simulink model "IPMSMTorqueBasedLoad_PQ"  (R2022a)
settings: Solver=FixedStepDiscrete  StartTime=0.0  StopTime=0.25  FixedStep=Ts  RelTol=1e-3  EnableMultiTasking=on
PreLoadFcn:
  | ee_ipmsm_torque_control_data;
  | Ts = 5e-6;
StopFcn:
  | ee_addSimlogTimeStamp(bdroot)
undefined symbols (not defined in the file or in its folder): Ld, Lq, p, psim, VDC_VECT
libraries: nesl_utility x13, fl_lib x9, ee_lib x5, eeTransforms x2, eePmsmCurrentController x1, simulink x1, eeGeneralControl x1, eePmsmCurrentReferenceGen x1, eePmsmTorqueEstimator x1, eePwmGeneratorTwoLevel x1, SignalEditorBlockLib x1
CloseFcn:
  | try,close(h1_ee_ipmsm_torque_control),end
  | clear h1_ee_ipmsm_torque_control
  | try,close(h2_ee_ipmsm_torque_control),end
  | clear h2_ee_ipmsm_torque_control
  | try,close(h3_ee_ipmsm_torque_control),end
  | clear h3_ee_ipmsm_torque_control
  | try,close(h4_ee_ipmsm_torque_control),end
  | clear h4_ee_ipmsm_torque_control
  | 
  | 
  | clear simlog_ee_ipmsm_torque_control
  | clear logsout_ee_ipmsm_torque_control
  | 
  | 
  | clear Pmax Tmax p psim Ld Lq L0 Rs Jm
  | clear Cdc Vnom V1 AH0
  | clear Ts fsw Tsi Kp_id Ki_id Kp_iq Ki_iq
  | clear numd_id dend_id numd_iq dend_iq
  | clear ID_MAP IQ_MAP RPM_VECT TQ_VECT VDC_VECT
Description:
  | IPMSM Torque Control
settings Model: Creator=The MathWorks, Inc.  LastModifiedBy=jvansick
settings SolverCC: AlgebraicLoopSolver=TrustRegion  MaxZcPerStep=1
settings DataIOCC: MaxDataPoints=210000  ReturnWorkspaceOutputs=off  SignalLoggingName=logsout_ee_ipmsm_torque_control
settings OptimizationCC: LifeSpan=inf
settings DebuggingCC: UnderspecifiedInitializationDetection=Classic  MergeDetectMultiDrivingBlocksExec=none  UnconnectedInputMsg=warning  UnconnectedOutputMsg=warning  UnconnectedLineMsg=warning  SFUnexpectedBacktrackingDiag=warning  SFNoUnconditionalDefaultTransitionDiag=warning  SFExecutionAtInitializationDiag=none  SFMachineParentedDataDiag=warning  ArithmeticOperatorsInVariantConditions=warning
settings SFSimCC: SimUseLocalCustomCode=off  CustomCodeUndefinedFunction=UseInterfaceOnly
settings RTWCC: RTWUseLocalCustomCode=off  DLArmComputeVersion=19.05
settings CodeAppCC: StateflowObjectComments=on
settings GRTTargetCC: TargetLangStandard=C89/C90 (ANSI)
settings ConfigComp: CovMetricSettings=dw  CovSaveCumulativeToWorkspaceVar=on  CovSaveSingleToWorkspaceVar=on  CovExternalEMLEnable=off
settings SimscapeCC: SimscapeNormalizeSystem=off  SimscapeLogType=all  SimscapeLogSimulationStatistics=on  SimscapeLogName=simlog_ee_ipmsm_torque_control  SimscapeLogDataHistory=210000

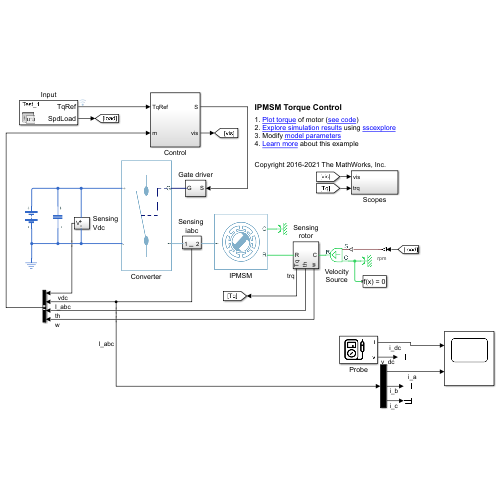
[thumbnail: Simulink's stored preview of the top-level diagram]
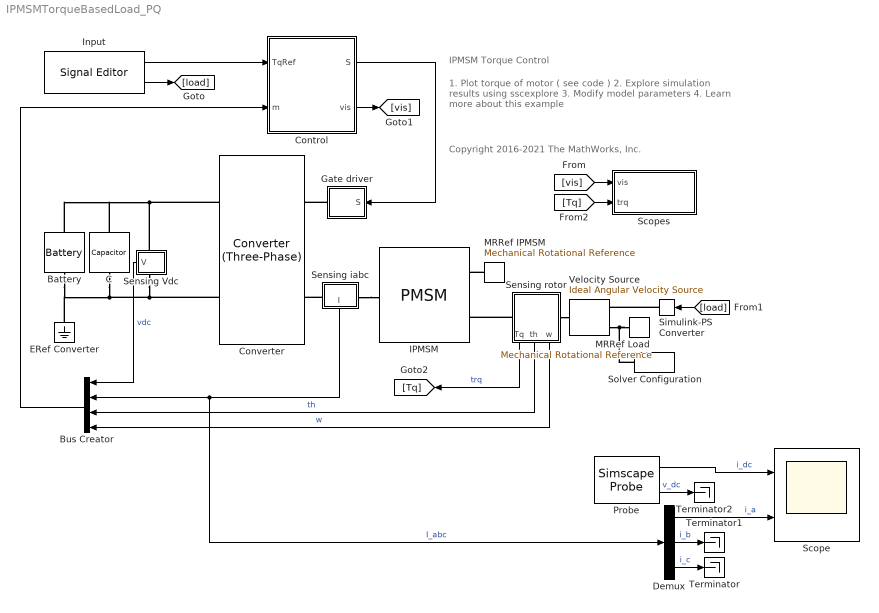
== system IPMSMTorqueBasedLoad_PQ ==
  note: IPMSM Torque Control
  note: 1. Plot torque of motor ( see code )
      | 2. Explore simulation results using sscexplore
      | 3. Modify model parameters
      | 4. Learn more about this example
  note: Copyright 2016-2021 The MathWorks, Inc.
  Battery : ee_lib/Sources/Battery  Vnom=Vnom V  prm_dir=1  R1_dis=2 Ohm  R1_ch=2 Ohm  R1=0.001 Ohm  prm_AH=1  AH=300 hr*A  V1=V1 V  AH1=100 hr*A  prm_R2=1  R2=2000 Ohm  prm_dyn=1  Rp1=0.005 Ohm  tau1=30 s  Rp2=0.005 Ohm  tau2=30 s  Rp3=0.005 Ohm  tau3=30 s  Rp4=0.005 Ohm  tau4=30 s  Rp5=0.005 Ohm  tau5=30 s  prm_fade=1  N_fade=100  AH_fade=45 hr*A  R1_fade=2.02 Ohm  R1_ch_fade=2.02 Ohm  V1_fade=10.35 V  prm_age=1  prm_age_OCV=1  OCV_age=0.9  SOC_age=60  delta_time_age_vec=[0] d  temperature_age_vec=[273] K  OCV_scaling_age=2.2134e6  OCV_offset_age=1.632e6  temp_exp_age=0.515833569 V  t_exp_age=0.75  i_specify=off  i_priority=None  i=0 A  i_nominal_specify=off  i_nominal_unit=A  i_nominal_value=1  v_specify=off  v_priority=None  v=0 V  v_nominal_specify=off  v_nominal_unit=V  v_nominal_value=1  charge_specify=on  charge_priority=High  charge=AH0 hr*A  charge_nominal_specify=off  charge_nominal_unit=hr*A  charge_nominal_value=1  num_cycles_specify=off  num_cycles_priority=High  num_cycles=0  num_cycles_nominal_specify=off  num_cycles_nominal_unit=1  num_cycles_nominal_value=1  Tmeas=298.15 K  Tmeas_age=298.15 K  Vnom_T2=12 V  R1_T2=2.2 Ohm  R1_T2_dis=2.2 Ohm  R1_T2_ch=2.2 Ohm  V1_T2=11.4 V  R2_T2=2200 Ohm  Rp1_T2=0.005 Ohm  tau1_T2=30 s  Rp2_T2=0.005 Ohm  tau2_T2=30 s  Rp3_T2=0.005 Ohm  tau3_T2=30 s  Rp4_T2=0.005 Ohm  tau4_T2=30 s  Rp5_T2=0.005 Ohm  tau5_T2=30 s  Tmeas2=273.15 K  thermal_mass=30000 J/K  temperature_specify=off  temperature_priority=High  temperature=298.15 K  temperature_nominal_specify=off  temperature_nominal_unit=K  temperature_nominal_value=1
  Bus Creator : BusCreator  Inputs=4
  C : fl_lib/Electrical/Electrical Elements/Capacitor  c=Cdc F  r=1e-6 Ohm  g=0 1/Ohm  i_specify=off  i_priority=None  i=0 A  i_nominal_specify=off  i_nominal_unit=A  i_nominal_value=1  v_specify=off  v_priority=None  v=0 V  v_nominal_specify=off  v_nominal_unit=V  v_nominal_value=1  vc_specify=on  vc_priority=None  vc=Vnom V  vc_nominal_specify=off  vc_nominal_unit=V  vc_nominal_value=1
      settings: SourceProductBaseCode=PW,SS,VE
  Control : Subsystem
  Converter : ee_lib/Semiconductors & Converters/Converters/Converter (Three-Phase)  port_option=ee.enum.threePhasePort.composite  device_type=3  Vf=0.8 V  Ron=0.001 Ohm  Rds=0.001 Ohm  Goff=1e-5 1/Ohm  Vgt=1 V  Vgt_off=-1 V  Ih=1 A  Vth=0.5 V  diode_param=2  diode_Vf=0.8 V  diode_Ron=0.001 Ohm  diode_Goff=1e-5 1/Ohm  diode_C=50 nF  diode_iRM=-235 A  diode_iF=300 A  diode_idot=-50 A/us  diode_trr_param=1  diode_trr_factor=3  diode_trr=15 us  diode_Qrr=1.5e+3 s*uA  snubber_type=0  Cs=1e-7 F  Rs=0.1 Ohm
      settings: SourceProductBaseCode=PS
  Demux : Demux  Outputs=3
  ERef Converter : fl_lib/Electrical/Electrical Elements/Electrical Reference
      settings: SourceProductBaseCode=PW,SS,VE
  Gate driver : Subsystem
  IPMSM : ee_lib/Electromechanical/Permanent Magnet/PMSM  port_option=ee.enum.threePhasePort.composite  winding_type=ee.enum.statorconnection.wye  machine_param=ee.enum.pmsm.parameterization.constant  nPolePairs=p  pmflux_param=ee.enum.pmflux.fluxlinkage  pm_flux_linkage=psim Wb  torque_constant=0.18 N*m/A  back_emf_constant=0.18 V/(rad/s)  stator_param=ee.enum.statorparam.LdLqL0  Ld=Ld H  Lq=Lq H  idVec=[-200, 0, 200] A  iqVec=[-200, 0, 200] A  LdMatrix=0.0002 * ones(3, 3) H  LqMatrix=0.0002 * ones(3, 3) H  PmMatrix=0.1 * ones(3, 3) Wb  ktMatrix=0.18 * ones(3, 3) N*m/A  keMatrix=0.18 * ones(3, 3) V/(rad/s)  L0=L0 H  Ls=0.0002 H  Lm=0.00002 H  Ms=0.00002 H  Rs=Rs Ohm  zero_sequence=ee.enum.park.zerosequence.exclude  axes_param=ee.enum.rotorangle.qaxis  loss_param=ee.enum.ironloss.none  losses_oc=[0, 0, 0] W  losses_sc=[0, 0, 0] W  f_losses=60 Hz  Isc_losses=95 A  J=0 kg*m^2  lam=0 N*m/(rad/s)  i_d_specify=off  i_d_priority=None  i_d=0 A  i_d_nominal_specify=off  i_d_nominal_unit=A  i_d_nominal_value=1  i_q_specify=off  i_q_priority=None  i_q=0 A  i_q_nominal_specify=off  i_q_nominal_unit=A  i_q_nominal_value=1  torque_specify=off  torque_priority=None  torque=0 N*m  torque_nominal_specify=off  torque_nominal_unit=N*m  torque_nominal_value=1  angular_velocity_specify=on  angular_velocity_priority=None  angular_velocity=0 rad/s  angular_velocity_nominal_specify=off  angular_velocity_nominal_unit=rpm  angular_velocity_nominal_value=1  angular_position_specify=on  angular_position_priority=High  angular_position=0 rad  angular_position_nominal_specify=off  angular_position_nominal_unit=deg  angular_position_nominal_value=1  alpha=3.93e-3 1/K  alpha_flux=-0.001 1/K  Tmeas=298.15 K  stator_thermal_mass=100 J/K  rotor_thermal_mass=200 J/K  Rm_percent_rotor=90  Rd_percent_rotor=30  temperatureA_specify=off  temperatureA_priority=High  temperatureA=25 degC  temperatureA_nominal_specify=off  temperatureA_nominal_unit=degC  temperatureA_nominal_value=1  temperatureB_specify=off  temperatureB_priority=High  temperatureB=25 degC  temperatureB_nominal_specify=off  temperatureB_nominal_unit=degC  temperatureB_nominal_value=1  temperatureC_specify=off  temperatureC_priority=High  temperatureC=25 degC  temperatureC_nominal_specify=off  temperatureC_nominal_unit=degC  temperatureC_nominal_value=1  temperatureR_specify=off  temperatureR_priority=High  temperatureR=25 degC  temperatureR_nominal_specify=off  temperatureR_nominal_unit=degC  temperatureR_nominal_value=1
      settings: InternalSimscapePortConfiguration="{\"Bottom\":[],\"Left\":[{\"id\":\"N\",\"label\":\"~\",\"type\":\"foundation.electrical.three_phase\"}],\"Right\":[{\"id\":\"R\",\"label\":\"R\",\"type\":\"foundation.mechanical.rotational.rotational\"},{\"id\":\"C\",\"label\":\"C\",\"type\":\"foundation.mechanical.rotational.rotational\"}],\"Top\":[]}"
  Input : SignalEditorBlockLib/Signal Editor  FileName=ee_ipmsm_torque_control_Input.mat  ActiveScenario=Test_1  ActiveSignal=TqRef  IsBus=off  OutputBusObjectStr=Bus: BusObject  SampleTime=0  Interpolate=off  ZeroCross=off  OutputAfterFinalValue=Setting to zero  Unit=inherit  PreserveSignalName=on
  MRRef IPMSM : fl_lib/Mechanical/Rotational Elements/Mechanical Rotational Reference
      settings: SourceProductBaseCode=PW,SS,VE
  MRRef Load : fl_lib/Mechanical/Rotational Elements/Mechanical Rotational Reference
      settings: SourceProductBaseCode=PW,SS,VE
  Probe : SimscapeProbe  BoundBlock=1058  Variables={i, v}
  Scope : Scope  NumInputPorts=2
  Scopes : Subsystem
      settings: PortSchema="{\"entries\":[{\"content\":{\"sides\":[{\"content\":{\"connectorIds\":[]},\"type\":\"ConnectorPlacement.EquallySpacedRectSide\",\"uuid\":\"a560794c-8dec-4526-a26c-129716e1b993\"},{\"content\":{\"connectorIds\":[\"In1\",\"In2\"],\"side\":\"RIGHT\"},\"type\":\"ConnectorPlacement.EquallySpacedRectSide\",\"uuid\":\"247ce755-40a5-4621-9d40-790612a7d15c\"},{\"content\":{\"connectorIds\":[],\"side\":\"TOP\"},\"type\":\"ConnectorPlacement.EquallySpacedRectSide\",\"uuid\":\"3a3e49bb-cf70-44be-b36a-46c371f23d10\"}]},\"type\":\"ConnectorPlacement.EquallySpacedConnector\",\"uuid\":\"881be24b-a5bc-43c9-adfc-ce8dee76105e\"}],\"packageUris\":[\"http://schema.mathworks.com/mf0/Connector/R2020b\"],\"version\":\"1.0\"}"
  Sensing Vdc : Subsystem
      settings: PortSchema="{\"entries\":[{\"content\":{\"sides\":[{\"content\":{\"connectorIds\":[\"LConn1\"]},\"type\":\"ConnectorPlacement.EquallySpacedRectSide\",\"uuid\":\"bc3757cc-4537-444e-89af-7b7d8c8c1fa7\"},{\"content\":{\"connectorIds\":[\"RConn1\"],\"side\":\"RIGHT\"},\"type\":\"ConnectorPlacement.EquallySpacedRectSide\",\"uuid\":\"908bf4c4-26f6-4d8a-bcf8-68236027f5f8\"},{\"content\":{\"connectorIds\":[\"Out1\"],\"side\":\"TOP\"},\"type\":\"ConnectorPlacement.EquallySpacedRectSide\",\"uuid\":\"33f228db-ba47-4718-96dc-a72de309ae8c\"},{\"content\":{\"connectorIds\":[],\"side\":\"BOTTOM\"},\"type\":\"ConnectorPlacement.EquallySpacedRectSide\",\"uuid\":\"d9b66c7e-0954-4c47-8bcc-77bf13ff573c\"}]},\"type\":\"ConnectorPlacement.EquallySpacedConnector\",\"uuid\":\"345f3578-0572-4e64-b2f3-84728129a12d\"}],\"packageUris\":[\"http://schema.mathworks.com/mf0/Connector/R2020b\"],\"version\":\"1.0\"}"
  Sensing rotor : Subsystem
      settings: PortSchema="{\"entries\":[{\"content\":{\"sides\":[{\"content\":{\"connectorIds\":[\"LConn1\"]},\"type\":\"ConnectorPlacement.EquallySpacedRectSide\",\"uuid\":\"bc3757cc-4537-444e-89af-7b7d8c8c1fa7\"},{\"content\":{\"connectorIds\":[\"RConn1\"],\"side\":\"RIGHT\"},\"type\":\"ConnectorPlacement.EquallySpacedRectSide\",\"uuid\":\"908bf4c4-26f6-4d8a-bcf8-68236027f5f8\"},{\"content\":{\"connectorIds\":[],\"side\":\"TOP\"},\"type\":\"ConnectorPlacement.EquallySpacedRectSide\",\"uuid\":\"33f228db-ba47-4718-96dc-a72de309ae8c\"},{\"content\":{\"connectorIds\":[\"Out1\",\"Out2\",\"Out3\"],\"side\":\"BOTTOM\"},\"type\":\"ConnectorPlacement.EquallySpacedRectSide\",\"uuid\":\"5b763560-fcc9-460b-9ba7-46235112184c\"}]},\"type\":\"ConnectorPlacement.EquallySpacedConnector\",\"uuid\":\"345f3578-0572-4e64-b2f3-84728129a12d\"}],\"packageUris\":[\"http://schema.mathworks.com/mf0/Connector/R2020b\"],\"version\":\"1.0\"}"
  Sensing iabc : Subsystem
      settings: PortSchema="{\"entries\":[{\"content\":{\"sides\":[{\"content\":{\"connectorIds\":[\"LConn1\"]},\"type\":\"ConnectorPlacement.EquallySpacedRectSide\",\"uuid\":\"bc3757cc-4537-444e-89af-7b7d8c8c1fa7\"},{\"content\":{\"connectorIds\":[\"RConn1\"],\"side\":\"RIGHT\"},\"type\":\"ConnectorPlacement.EquallySpacedRectSide\",\"uuid\":\"908bf4c4-26f6-4d8a-bcf8-68236027f5f8\"},{\"content\":{\"connectorIds\":[],\"side\":\"TOP\"},\"type\":\"ConnectorPlacement.EquallySpacedRectSide\",\"uuid\":\"33f228db-ba47-4718-96dc-a72de309ae8c\"},{\"content\":{\"connectorIds\":[\"Out1\"],\"side\":\"BOTTOM\"},\"type\":\"ConnectorPlacement.EquallySpacedRectSide\",\"uuid\":\"3b1d40a5-3c80-431c-8111-df754e0c502b\"}]},\"type\":\"ConnectorPlacement.EquallySpacedConnector\",\"uuid\":\"345f3578-0572-4e64-b2f3-84728129a12d\"}],\"packageUris\":[\"http://schema.mathworks.com/mf0/Connector/R2020b\"],\"version\":\"1.0\"}"
  Simulink-PS Converter : nesl_utility/Simulink-PS Converter  PhysicalDomain=network_engine_domain  SubClassName=ps_input  LeftPortType=input  RightPortType=output  PseudoPeriodic=off  Frequencies=[]  NoiseDistribution=none  NoiseParameters=[]  Unit=rpm  AffineConversion=off  FilteringAndDerivatives=zero  SimscapeFilterOrder=1  InputFilterTimeConstant=0.001  UdotUserProvided=1
      settings: SourceProductBaseCode=SS,PW,VE
  Solver Configuration : nesl_utility/Solver Configuration  PhysicalDomain=network_engine_domain  SubClassName=solver  LeftPortType=input  RightPortType=generic  Tones=[]  Harmonics=[]  SimulateNoise=off  Profile=off  UseLocalSampling=off  EnableSwitchedLinearOptims=on  FrequencyDomain=off  UseCCode=off  RelTol=0.001  AbsTol=1e-06  MinStep=1e-09  ToWorkspace=off  RevertToSquareIcSolve=off  NumHomotopyIterations=100  PhasorMode=off  PhasorModeNumHarmonics=1  IndexReductionMethod=DerivativeReplacement  DoDC=off  ResidualTolerance=1e-9  UseLocalSolver=on  LocalSolverChoice=NE_BACKWARD_EULER_ADVANCER  LocalSolverSampleTime=Ts  DoFixedCost=on  MaxNonlinIter=5  MaxModeIter=2  ComputeImpulses=off  ImpulseIterations=2  LinearAlgebra=auto  LinearAlgebraNumThread=0  EquationFormulation=NE_TIME_EF  DelaysMemoryBudget=1024  AutomaticFiltering=on  FilteringTimeConstant=0.001  PartitionStorageMethod=AS_NEEDED  PartitionMemoryBudget=1024  PartitionMethod=FAST
      settings: SourceProductBaseCode=SS,PW,VE
  Terminator : Terminator
  Terminator1 : Terminator
  Terminator2 : Terminator
  Velocity Source : fl_lib/Mechanical/Mechanical Sources/Ideal Angular Velocity Source
      settings: SourceProductBaseCode=PW,SS,VE
  wires:
  [load] -> Simulink-PS Converter/1
  Input/2 -> [load]
  [vis] -> Scopes/1(vis)
  Bus Creator/1 -> Control/2(m)
  Input/1 -> Control/1(TqRef)
  Control/1(S) -> Gate driver/1(S)
  Control/2(vis) -> [vis]
  Sensing Vdc/1(V) -> Bus Creator/1  "vdc"
  Sensing iabc/1(I) -> Demux/1, Bus Creator/2  "I_abc"
  Sensing rotor/2(th) -> Bus Creator/3  "th"
  Sensing rotor/3(w) -> Bus Creator/4  "w"
  Sensing rotor/1(Tq) -> [Tq]  "trq"
  [Tq] -> Scopes/2(trq)
  Probe/1 -> Scope/1  "i_dc"
  Demux/1 -> Scope/2  "i_a"
  Demux/3 -> Terminator/1  "i_c"
  Demux/2 -> Terminator1/1  "i_b"
  Probe/2 -> Terminator2/1  "v_dc"
  connections:
  Velocity Source/RConn2 -- Solver Configuration/RConn1 -- MRRef Load/LConn1
  Converter/RConn2 -- Sensing Vdc/RConn1 -- Battery/RConn1 -- ERef Converter/LConn1 -- C/RConn1
  Converter/RConn1 -- Battery/LConn1 -- C/LConn1 -- Sensing Vdc/LConn1
  Gate driver/RConn1 -- Converter/LConn1
  Simulink-PS Converter/RConn1 -- Velocity Source/RConn1
  Sensing iabc/LConn1 -- Converter/LConn2
  Sensing iabc/RConn1 -- IPMSM/LConn1
  MRRef IPMSM/LConn1 -- IPMSM/RConn2
  Sensing rotor/LConn1 -- IPMSM/RConn1
  Sensing rotor/RConn1 -- Velocity Source/LConn1

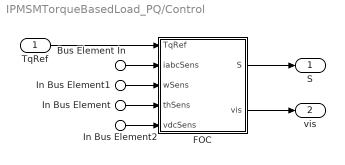
== system IPMSMTorqueBasedLoad_PQ/Control ==
  TqRef : Inport
  Bus Element In : Inport  Port=2  PortName=m  Element=I_abc
  In Bus Element : Inport  Port=2  PortName=m  Element=th
  In Bus Element1 : Inport  Port=2  PortName=m  Element=w
  In Bus Element2 : Inport  Port=2  PortName=m  Element=vdc
  FOC : Subsystem
  S : Outport
  vis : Outport  Port=2
  wires:
  FOC/1(S) -> S/1
  TqRef/1 -> FOC/1(TqRef)
  FOC/2(vis) -> vis/1
  Bus Element In/1 -> FOC/2(iabcSens)
  In Bus Element2/1 -> FOC/5(vdcSens)
  In Bus Element1/1 -> FOC/3(wSens)
  In Bus Element/1 -> FOC/4(thSens)

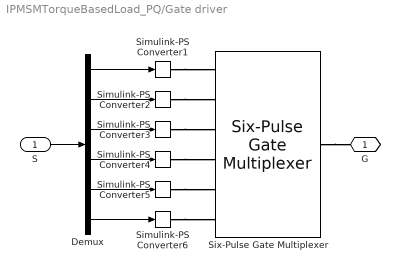
== system IPMSMTorqueBasedLoad_PQ/Gate driver ==
  S : Inport
  Demux : Demux  Outputs=6
  Simulink-PS Converter{1..6} (6 alike) : nesl_utility/Simulink-PS Converter  PhysicalDomain=network_engine_domain  SubClassName=ps_input  LeftPortType=input  RightPortType=output  PseudoPeriodic=off  Frequencies=[]  NoiseDistribution=none  NoiseParameters=[]  Unit=1  AffineConversion=off  FilteringAndDerivatives=zero  SimscapeFilterOrder=1  InputFilterTimeConstant=0.001  UdotUserProvided=1
      settings: SourceProductBaseCode=SS,PW,VE
  Six-Pulse Gate Multiplexer : ee_lib/Semiconductors & Converters/Converters/Six-Pulse Gate Multiplexer  port_option=ee.enum.controlport.ps
      settings: SourceProductBaseCode=PS
  G : PMIOPort  Side=Right
  wires:
  Demux/1 -> Simulink-PS Converter1/1
  S/1 -> Demux/1
  Demux/5 -> Simulink-PS Converter5/1
  Demux/6 -> Simulink-PS Converter6/1
  Demux/4 -> Simulink-PS Converter4/1
  Demux/3 -> Simulink-PS Converter3/1
  Demux/2 -> Simulink-PS Converter2/1
  connections:
  Six-Pulse Gate Multiplexer/RConn1 -- G/RConn1
  Simulink-PS Converter1/RConn1 -- Six-Pulse Gate Multiplexer/LConn1
  Simulink-PS Converter5/RConn1 -- Six-Pulse Gate Multiplexer/LConn5
  Simulink-PS Converter6/RConn1 -- Six-Pulse Gate Multiplexer/LConn6
  Simulink-PS Converter2/RConn1 -- Six-Pulse Gate Multiplexer/LConn2
  Simulink-PS Converter3/RConn1 -- Six-Pulse Gate Multiplexer/LConn3
  Simulink-PS Converter4/RConn1 -- Six-Pulse Gate Multiplexer/LConn4

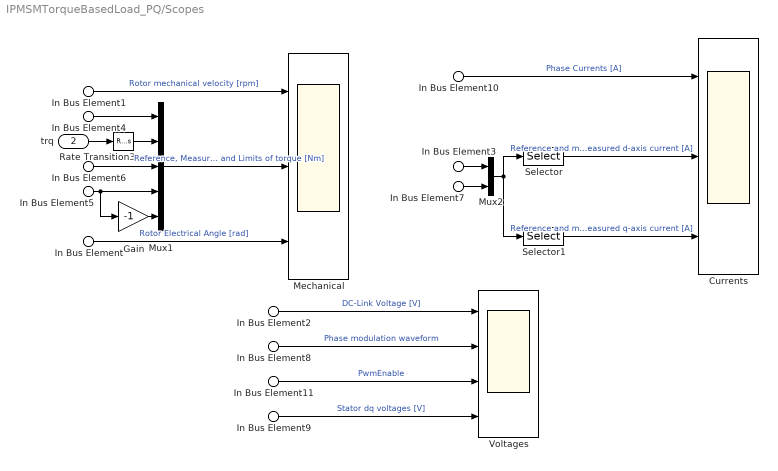
== system IPMSMTorqueBasedLoad_PQ/Scopes ==
  In Bus Element1 : Inport  PortName=vis  Element=Spd
  In Bus Element : Inport  PortName=vis  Element=AngElec
  In Bus Element2 : Inport  PortName=vis  Element=vdc
  In Bus Element3 : Inport  PortName=vis  Element=idqRef
  In Bus Element4 : Inport  PortName=vis  Element=TqRef
  In Bus Element5 : Inport  PortName=vis  Element=TqLim
  In Bus Element6 : Inport  PortName=vis  Element=TqEstim
  In Bus Element7 : Inport  PortName=vis  Element=idq
  In Bus Element8 : Inport  PortName=vis  Element=ModWave
  In Bus Element9 : Inport  PortName=vis  Element=vdq
  In Bus Element10 : Inport  PortName=vis  Element=Iabc
  In Bus Element11 : Inport  PortName=vis  Element=PwmEna
  trq : Inport  Port=2
  Currents : Scope  NumInputPorts=3
  Gain : Gain  Gain=-1
  Mechanical : Scope  NumInputPorts=3
  Mux1 : Mux  Inputs=5
  Mux2 : Mux  Inputs=2
  Rate Transition3 : RateTransition
  Selector : Selector  InputPortWidth=4  IndexOptions=Index vector (dialog)  Indices=[1 3]  OutputSizes=1
  Selector1 : Selector  InputPortWidth=4  IndexOptions=Index vector (dialog)  Indices=[2 4]  OutputSizes=1
  Voltages : Scope  NumInputPorts=4
  wires:
  In Bus Element1/1 -> Mechanical/1  "Rotor mechanical velocity [rpm]"
  Mux1/1 -> Mechanical/2  "Reference, Measured, Estim and Limits of torque [Nm]"
  In Bus Element4/1 -> Mux1/1
  In Bus Element/1 -> Mechanical/3  "Rotor Electrical Angle [rad]"
  In Bus Element9/1 -> Voltages/4  "Stator dq voltages [V]"
  In Bus Element5/1 -> Gain/1, Mux1/4
  In Bus Element8/1 -> Voltages/2  "Phase modulation waveform"
  In Bus Element2/1 -> Voltages/1  "DC-Link Voltage [V]"
  In Bus Element10/1 -> Currents/1  "Phase Currents [A]"
  Selector1/1 -> Currents/3  "Reference and measured q-axis current [A]"
  In Bus Element3/1 -> Mux2/1
  Selector/1 -> Currents/2  "Reference and measured d-axis current [A]"
  Mux2/1 -> Selector1/1, Selector/1
  In Bus Element7/1 -> Mux2/2
  Gain/1 -> Mux1/5
  In Bus Element6/1 -> Mux1/3
  Rate Transition3/1 -> Mux1/2
  In Bus Element11/1 -> Voltages/3  "PwmEnable"
  trq/1 -> Rate Transition3/1

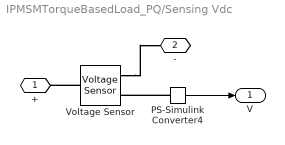
== system IPMSMTorqueBasedLoad_PQ/Sensing Vdc ==
  PS-Simulink Converter4 : nesl_utility/PS-Simulink Converter  PhysicalDomain=network_engine_domain  SubClassName=ps_output  LeftPortType=input  RightPortType=output  PseudoPeriodic=off  Frequencies=[]  VectorFormat=1-D array  Unit=V  AffineConversion=off
      settings: SourceProductBaseCode=SS,PW,VE
  Voltage Sensor : fl_lib/Electrical/Electrical Sensors/Voltage Sensor
      settings: SourceProductBaseCode=PW,SS,VE
  + : PMIOPort  Side=Left
  - : PMIOPort  Port=2  Side=Right
  V : Outport
  wires:
  PS-Simulink Converter4/1 -> V/1
  connections:
  Voltage Sensor/LConn1 -- +/RConn1
  Voltage Sensor/RConn2 -- -/RConn1
  PS-Simulink Converter4/LConn1 -- Voltage Sensor/RConn1

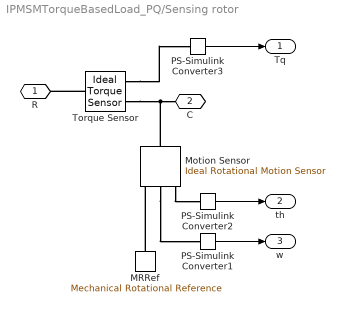
== system IPMSMTorqueBasedLoad_PQ/Sensing rotor ==
  MRRef : fl_lib/Mechanical/Rotational Elements/Mechanical Rotational Reference
      settings: SourceProductBaseCode=PW,SS,VE
  Motion Sensor : fl_lib/Mechanical/Mechanical Sensors/Ideal Rotational Motion Sensor  wrap_angle=simscape.enum.onoff.off  offset=0 deg
      settings: SourceProductBaseCode=PW,SS,VE
  PS-Simulink Converter1 : nesl_utility/PS-Simulink Converter  PhysicalDomain=network_engine_domain  SubClassName=ps_output  LeftPortType=input  RightPortType=output  PseudoPeriodic=off  Frequencies=[]  VectorFormat=1-D array  Unit=rad/s  AffineConversion=off
      settings: SourceProductBaseCode=SS,PW,VE
  PS-Simulink Converter2 : nesl_utility/PS-Simulink Converter  PhysicalDomain=network_engine_domain  SubClassName=ps_output  LeftPortType=input  RightPortType=output  PseudoPeriodic=off  Frequencies=[]  VectorFormat=1-D array  Unit=rad  AffineConversion=off
      settings: SourceProductBaseCode=SS,PW,VE
  PS-Simulink Converter3 : nesl_utility/PS-Simulink Converter  PhysicalDomain=network_engine_domain  SubClassName=ps_output  LeftPortType=input  RightPortType=output  PseudoPeriodic=off  Frequencies=[]  VectorFormat=1-D array  Unit=N*m  AffineConversion=off
      settings: SourceProductBaseCode=SS,PW,VE
  Torque Sensor : fl_lib/Mechanical/Mechanical Sensors/Ideal Torque Sensor
      settings: SourceProductBaseCode=PW,SS,VE
  R : PMIOPort  Side=Left
  C : PMIOPort  Port=2  Side=Right
  Tq : Outport
  th : Outport  Port=2
  w : Outport  Port=3
  wires:
  PS-Simulink Converter3/1 -> Tq/1
  PS-Simulink Converter2/1 -> th/1
  PS-Simulink Converter1/1 -> w/1
  connections:
  Torque Sensor/RConn1 -- Motion Sensor/LConn1 -- C/RConn1
  Torque Sensor/RConn2 -- PS-Simulink Converter3/LConn1
  Torque Sensor/LConn1 -- R/RConn1
  Motion Sensor/RConn2 -- PS-Simulink Converter1/LConn1
  MRRef/LConn1 -- Motion Sensor/RConn1
  Motion Sensor/RConn3 -- PS-Simulink Converter2/LConn1

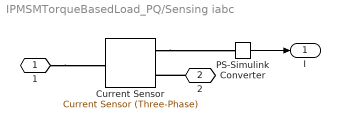
== system IPMSMTorqueBasedLoad_PQ/Sensing iabc ==
  Current Sensor : ee_lib/Sensors & Transducers/Current Sensor (Three-Phase)
  PS-Simulink Converter : nesl_utility/PS-Simulink Converter  PhysicalDomain=network_engine_domain  SubClassName=ps_output  LeftPortType=input  RightPortType=output  PseudoPeriodic=off  Frequencies=[]  VectorFormat=1-D array  Unit=A  AffineConversion=off
      settings: SourceProductBaseCode=SS,PW,VE
  1 : PMIOPort  Side=Left
  2 : PMIOPort  Port=2  Side=Right
  I : Outport
  wires:
  PS-Simulink Converter/1 -> I/1
  connections:
  1/RConn1 -- Current Sensor/LConn1
  2/RConn1 -- Current Sensor/RConn2
  Current Sensor/RConn1 -- PS-Simulink Converter/LConn1

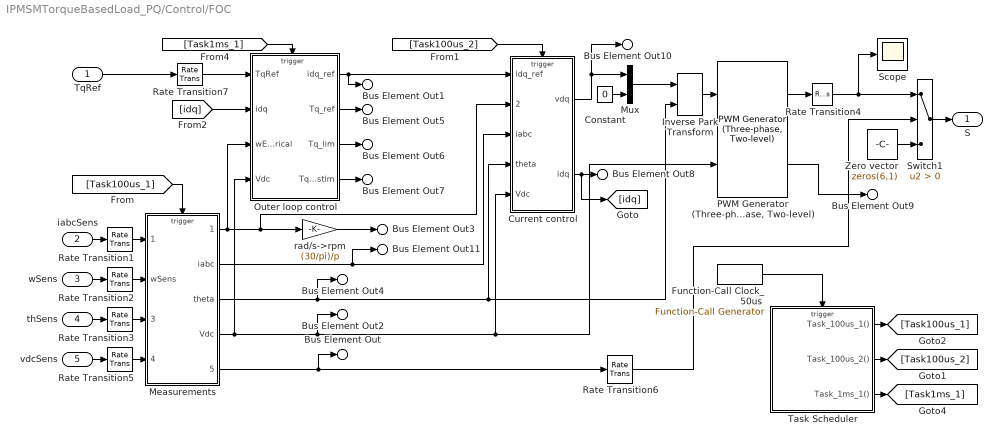
== system IPMSMTorqueBasedLoad_PQ/Control/FOC ==
  TqRef : Inport
  iabcSens : Inport  Port=2
  wSens : Inport  Port=3
  thSens : Inport  Port=4
  vdcSens : Inport  Port=5
  Constant : Constant  Value=0  SampleTime=-1
  Current control : Subsystem
  Function-Call Clock_50us : simulink/Ports & Subsystems/Function-Call Generator  sample_time=5e-5  numberOfIterations=1  DisallowWideOutput=off
  Inverse Park Transform : eeTransforms/Inverse Park Transform  AxisAlignment=Q-axis  PowerInvariant=off
  Measurements : Subsystem
  Mux : Mux  Inputs=2
  Outer loop control : Subsystem
  "PWM Generator (Three-phase, Two-level)" : eePwmGeneratorTwoLevel/PWM Generator (Three-phase, Two-level)  PWMMode=Continuous PWM (CPWM)  CPWMMode=SVM: space vector modulation  DPWMMode=60 DPWM: 60 degree discontinuous PWM  fsw=fsw  Ts=Ts
      settings: SourceProductBaseCode=PS
  Rate Transition{1..7} (7 alike) : RateTransition
  Scope : Scope
  Switch1 : Switch  Criteria=u2 > Threshold  SaturateOnIntegerOverflow=off  InputSameDT=off
  Task Scheduler : Stateflow chart  TreatAsAtomicUnit=on
  Zero vector : Constant  Value=zeros(6,1)
  rad/s->rpm : Gain  Gain=(30/pi)/p
  S : Outport  VectorParamsAs1DForOutWhenUnconnected=off
  Bus Element Out : Outport  Port=2  PortName=vis  Element=PwmEna
  Bus Element Out3 : Outport  Port=2  PortName=vis  Element=Spd
  Bus Element Out4 : Outport  Port=2  PortName=vis  Element=AngElec
  Bus Element Out2 : Outport  Port=2  PortName=vis  Element=vdc
  Bus Element Out1 : Outport  Port=2  PortName=vis  Element=idqRef
  Bus Element Out5 : Outport  Port=2  PortName=vis  Element=TqRef
  Bus Element Out6 : Outport  Port=2  PortName=vis  Element=TqLim
  Bus Element Out7 : Outport  Port=2  PortName=vis  Element=TqEstim
  Bus Element Out8 : Outport  Port=2  PortName=vis  Element=idq
  Bus Element Out9 : Outport  Port=2  PortName=vis  Element=ModWave
  Bus Element Out10 : Outport  Port=2  PortName=vis  Element=vdq
  Bus Element Out11 : Outport  Port=2  PortName=vis  Element=Iabc
  wires:
  [Task100us_2] -> Current control/Trigger
  [Task1ms_1] -> Outer loop control/Trigger
  Current control/1(vdq) -> Bus Element Out10/1, Mux/1
  Measurements/2(iabc) -> Bus Element Out11/1, Current control/3(iabc)
  Measurements/3(theta) -> Bus Element Out4/1, Inverse Park Transform/2, Current control/4(theta)
  "PWM Generator (Three-phase, Two-level)"/1 -> Rate Transition4/1
  Inverse Park Transform/1 -> "PWM Generator (Three-phase, Two-level)"/1
  iabcSens/1 -> Rate Transition1/1
  wSens/1 -> Rate Transition2/1
  thSens/1 -> Rate Transition3/1
  vdcSens/1 -> Rate Transition5/1
  Outer loop control/1(idq_ref) -> Bus Element Out1/1, Current control/1(idq_ref)
  "PWM Generator (Three-phase, Two-level)"/2 -> Bus Element Out9/1
  Rate Transition1/1 -> Measurements/1(iabcSens)
  Rate Transition2/1 -> Measurements/2(wSens)
  Rate Transition3/1 -> Measurements/3(thSens)
  Rate Transition5/1 -> Measurements/4(VdcSens)
  Measurements/4(Vdc) -> Bus Element Out2/1, Current control/5(Vdc), "PWM Generator (Three-phase, Two-level)"/2, Outer loop control/4(Vdc)
  Function-Call Clock_50us/1 -> Task Scheduler/Trigger
  Task Scheduler/3(Task_1ms_1()) -> [Task1ms_1]
  Task Scheduler/2(Task_100us_2()) -> [Task100us_2]
  Task Scheduler/1(Task_100us_1()) -> [Task100us_1]
  Outer loop control/2(Tq_ref) -> Bus Element Out5/1
  Measurements/1(wElectrical) -> Current control/2(wElectrical), rad/s->rpm/1, Outer loop control/3(wElectrical)
  rad/s->rpm/1 -> Bus Element Out3/1
  Outer loop control/3(Tq_lim) -> Bus Element Out6/1
  Rate Transition7/1 -> Outer loop control/1(TqRef)
  TqRef/1 -> Rate Transition7/1
  Outer loop control/4(Tq_estim) -> Bus Element Out7/1
  [idq] -> Outer loop control/2(idq)
  Switch1/1 -> S/1
  Rate Transition4/1 -> Switch1/1, Scope/1
  Measurements/5(PwmEnable) -> Bus Element Out/1, Rate Transition6/1
  Zero vector/1 -> Switch1/3
  Rate Transition6/1 -> Switch1/2
  Current control/2(idq) -> [idq], Bus Element Out8/1
  [Task100us_1] -> Measurements/Trigger
  Constant/1 -> Mux/2
  Mux/1 -> Inverse Park Transform/1

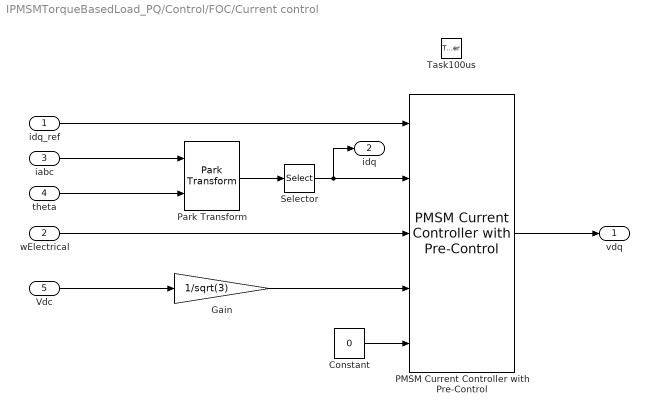
== system IPMSMTorqueBasedLoad_PQ/Control/FOC/Current control ==
  idq_ref : Inport
  wElectrical : Inport  Port=2
  iabc : Inport  Port=3
  theta : Inport  Port=4
  Vdc : Inport  Port=5
  Task100us : TriggerPort  TriggerType=function-call  VariantControl=Variant  PortDimensions=1
  Constant : Constant  Value=0  SampleTime=-1
  Gain : Gain  Gain=1/sqrt(3)
  PMSM Current Controller with Pre-Control : eePmsmCurrentController/PMSM Current Controller with Pre-Control  Kp_id=Kp_id  Ki_id=Ki_id  Kaw_id=1  Kp_iq=Kp_iq  Ki_iq=Ki_iq  Kaw_iq=1  Ts=-1  Tsd=Tsi  AxisPrio=Q-axis  ActZC=on  ActFF=on  idVect=[-200, 0, 200]  iqVect=[-200, 0, 200]  LdMatrix=Ld * ones(3, 3)  LqMatrix=Lq * ones(3, 3)  psimMatrix=psim * ones(3, 3)
      settings: SourceProductBaseCode=PS
  Park Transform : eeTransforms/Park Transform  AxisAlignment=Q-axis  PowerInvariant=off
  Selector : Selector  InputPortWidth=3  IndexOptions=Index vector (dialog)  Indices=[1 2]  OutputSizes=1
  vdq : Outport  VectorParamsAs1DForOutWhenUnconnected=off
  idq : Outport  Port=2  VectorParamsAs1DForOutWhenUnconnected=off
  wires:
  Park Transform/1 -> Selector/1
  Gain/1 -> PMSM Current Controller with Pre-Control/4
  Selector/1 -> idq/1, PMSM Current Controller with Pre-Control/2
  Constant/1 -> PMSM Current Controller with Pre-Control/5
  PMSM Current Controller with Pre-Control/1 -> vdq/1
  wElectrical/1 -> PMSM Current Controller with Pre-Control/3
  idq_ref/1 -> PMSM Current Controller with Pre-Control/1
  theta/1 -> Park Transform/2
  iabc/1 -> Park Transform/1
  Vdc/1 -> Gain/1

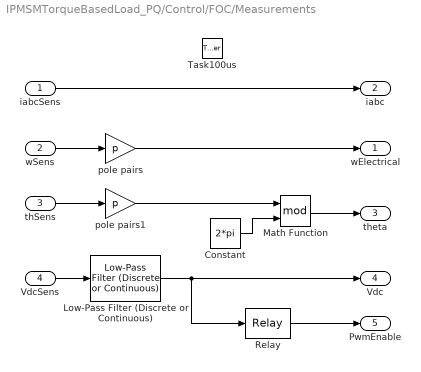
== system IPMSMTorqueBasedLoad_PQ/Control/FOC/Measurements ==
  iabcSens : Inport
  wSens : Inport  Port=2
  thSens : Inport  Port=3
  VdcSens : Inport  Port=4
  Task100us : TriggerPort  TriggerType=function-call  VariantControl=Variant  PortDimensions=1
  Constant : Constant  Value=2*pi  SampleTime=-1
  Low-Pass Filter (Discrete or Continuous) : eeGeneralControl/Low-Pass Filter (Discrete or Continuous)  K=1  T=0.005  B=inf  A=-inf  init_option=Inherited from block input  x0=0  Ts=-1
  Math Function : Math  Operator=mod  SignedPower=on
  Relay : Relay  OnSwitchValue=VDC_VECT(1)  OffSwitchValue=0.5*VDC_VECT(1)
  pole pairs : Gain  Gain=p
  pole pairs1 : Gain  Gain=p
  wElectrical : Outport  VectorParamsAs1DForOutWhenUnconnected=off
  iabc : Outport  Port=2  VectorParamsAs1DForOutWhenUnconnected=off
  theta : Outport  Port=3  VectorParamsAs1DForOutWhenUnconnected=off
  Vdc : Outport  Port=4  VectorParamsAs1DForOutWhenUnconnected=off
  PwmEnable : Outport  Port=5  VectorParamsAs1DForOutWhenUnconnected=off
  wires:
  pole pairs/1 -> wElectrical/1
  VdcSens/1 -> Low-Pass Filter (Discrete or Continuous)/1
  thSens/1 -> pole pairs1/1
  wSens/1 -> pole pairs/1
  iabcSens/1 -> iabc/1
  pole pairs1/1 -> Math Function/1
  Constant/1 -> Math Function/2
  Math Function/1 -> theta/1
  Relay/1 -> PwmEnable/1
  Low-Pass Filter (Discrete or Continuous)/1 -> Relay/1, Vdc/1

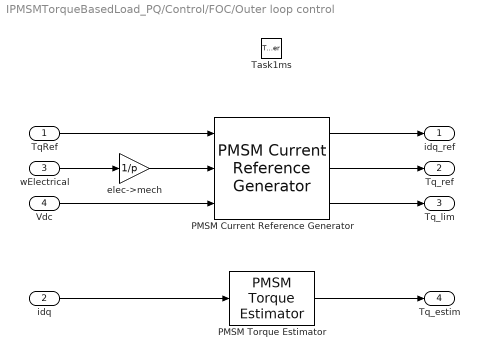
== system IPMSMTorqueBasedLoad_PQ/Control/FOC/Outer loop control ==
  TqRef : Inport
  idq : Inport  Port=2
  wElectrical : Inport  Port=3
  Vdc : Inport  Port=4
  Task1ms : TriggerPort  TriggerType=function-call  VariantControl=Variant  PortDimensions=1
  PMSM Current Reference Generator : eePmsmCurrentReferenceGen/PMSM Current Reference Generator  Vnom=Vnom  Pmax=Pmax  Tmax=Tmax  Ts=-1  RefType=Lookup-table based  rpmVec=RPM_VECT  TqVec=TQ_VECT  VdcVec=VDC_VECT  PWMMode=SVM: space vector modulation  ModFactor=1  idMatrix=ID_MAP  iqMatrix=IQ_MAP  p=8  psim=0.04  Ld=0.00024  Lq=0.00029  Rs=0.01  RefExpEnable=0
      settings: SourceProductBaseCode=PS
  PMSM Torque Estimator : eePmsmTorqueEstimator/PMSM Torque Estimator  ParamType=Constant parameters  p=p  idVect=[-200, 200]  iqVect=[-200, 200]  LdMatrix=0.0002 * ones(2, 2)  LqMatrix=0.0002 * ones(2, 2)  psimMatrix=0.04 * ones(2, 2)  Ld=Ld  Lq=Lq  psim=psim  Ts=-1
      settings: SourceProductBaseCode=PS
  elec->mech : Gain  Gain=1/p
  idq_ref : Outport  VectorParamsAs1DForOutWhenUnconnected=off
  Tq_ref : Outport  Port=2  VectorParamsAs1DForOutWhenUnconnected=off
  Tq_lim : Outport  Port=3  VectorParamsAs1DForOutWhenUnconnected=off
  Tq_estim : Outport  Port=4  VectorParamsAs1DForOutWhenUnconnected=off
  wires:
  wElectrical/1 -> elec->mech/1
  elec->mech/1 -> PMSM Current Reference Generator/2
  TqRef/1 -> PMSM Current Reference Generator/1
  Vdc/1 -> PMSM Current Reference Generator/3
  PMSM Current Reference Generator/1 -> idq_ref/1
  PMSM Current Reference Generator/2 -> Tq_ref/1
  PMSM Current Reference Generator/3 -> Tq_lim/1
  idq/1 -> PMSM Torque Estimator/1
  PMSM Torque Estimator/1 -> Tq_estim/1

== stateflow chart IPMSMTorqueBasedLoad_PQ/Control/FOC/Task Scheduler ==
  (default) -> (junction 23) : CLK_50us
  (junction 23) -> (junction 17)
  (junction 17) -> (junction 22) [order 2]
  (junction 17) -> (junction 22) [order 1] : [cnt%%2==0]{Task_100us_1;}
  (junction 22) -> (junction 18) [order 2]
  (junction 22) -> (junction 18) [order 1] : [cnt%%2==0]{Task_100us_2;}
  (junction 18) -> (junction 21) [order 1] : [cnt%%20==0]{Task_1ms_1;}
  (junction 18) -> (junction 21) [order 2]
  (junction 21) -> (junction 34) [order 2]
  (junction 21) -> (junction 16) [order 1] : [1]{cnt++;}
  data: cnt local int32
  events: Task_100us_1 output FUNCTION_CALL_EVENT; Task_100us_2 output FUNCTION_CALL_EVENT; Task_1ms_1 output FUNCTION_CALL_EVENT; CLK_50us input FUNCTION_CALL_EVENT
